simulink model "traffic_light_with_urgent_manger_B2B"  (R2020a)
settings: Solver=VariableStepAuto  StartTime=0.0  StopTime=10.0  RelTol=1e-3
libraries: pil_lib x1
settings Model: Creator=Administrator  LastModifiedBy=Administrator

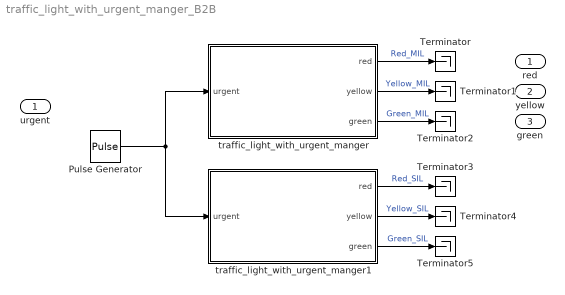
== system traffic_light_with_urgent_manger_B2B ==
  urgent : Inport
  Pulse Generator : DiscretePulseGenerator  PulseType=Time based  Period=10  PulseWidth=5
  Terminator{,1..5} (6 alike) : Terminator
  traffic_light_with_urgent_manger : Stateflow chart  TreatAsAtomicUnit=on
  traffic_light_with_urgent_manger1 : Subsystem  Tag=__SL_testing_harness_stub_  DialogController=pil_create_dialog  LoadFcn=|
      | try
      |    if ~strcmp(rtw.pil.getPILVersion, '9.8 (R2020a)_13')
      |       set_param(gcb, 'DialogController', '');
      |       set_param(gcb, 'DialogControllerArgs', '');
      |    end
      | catch e
      |       set_param(gcb, 'DialogController', '');
      |       set_param(gcb, 'DialogControllerArgs', '');
      | end
      mask help: PIL:pil:XILBlockMaskDesc
      mask Display: disp('SIL');
  red : Outport
  yellow : Outport  Port=2
  green : Outport  Port=3
  wires:
  Pulse Generator/1 -> traffic_light_with_urgent_manger1/1(urgent), traffic_light_with_urgent_manger/1(urgent)
  traffic_light_with_urgent_manger/1(red) -> Terminator/1  "Red_MIL"
  traffic_light_with_urgent_manger/2(yellow) -> Terminator1/1  "Yellow_MIL"
  traffic_light_with_urgent_manger/3(green) -> Terminator2/1  "Green_MIL"
  traffic_light_with_urgent_manger1/1(red) -> Terminator3/1  "Red_SIL"
  traffic_light_with_urgent_manger1/2(yellow) -> Terminator4/1  "Yellow_SIL"
  traffic_light_with_urgent_manger1/3(green) -> Terminator5/1  "Green_SIL"

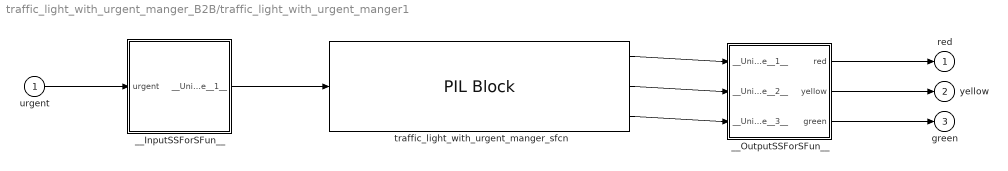
== system traffic_light_with_urgent_manger_B2B/traffic_light_with_urgent_manger1 ==
  urgent : Inport
  __InputSSForSFun__ : Subsystem
  __OutputSSForSFun__ : Subsystem
  traffic_light_with_urgent_manger_sfcn : pil_lib/PIL Block  SimulationMode=SIL  IsTopModelPIL=off  CodeDir=C:\Users\Administrator\Desktop\2020m\state_flow\1\traffic_light_with_urgent_manger\traffic_light_with_urgent_mange_ert_rtw  AnchorDir=C:\Users\Administrator\Desktop\2020m\state_flow\1\traffic_light_with_urgent_manger  ConfigName=Software-in-the-Loop (SIL)  XrelIsTopModelCode=on  XrelIsReusable=off  XrelDWorkNames={}  XrelDWorkTypes={}  XrelModelArgVals={}  XrelOrderedParamNames={}
      settings: SourceProductBaseCode=RT
  red : Outport
  yellow : Outport  Port=2
  green : Outport  Port=3
  wires:
  __OutputSSForSFun__/3(green) -> green/1
  __OutputSSForSFun__/2(yellow) -> yellow/1
  __OutputSSForSFun__/1(red) -> red/1
  traffic_light_with_urgent_manger_sfcn/3 -> __OutputSSForSFun__/3(__UniqueInportName__3__)
  traffic_light_with_urgent_manger_sfcn/2 -> __OutputSSForSFun__/2(__UniqueInportName__2__)
  traffic_light_with_urgent_manger_sfcn/1 -> __OutputSSForSFun__/1(__UniqueInportName__1__)
  __InputSSForSFun__/1(__UniqueOutportName__1__) -> traffic_light_with_urgent_manger_sfcn/1
  urgent/1 -> __InputSSForSFun__/1(urgent)

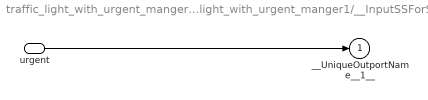
== system traffic_light_with_urgent_manger_B2B/traffic_light_with_urgent_manger1/__InputSSForSFun__ ==
  urgent : Inport
  __UniqueOutportName__1__ : Outport
  wires:
  urgent/1 -> __UniqueOutportName__1__/1

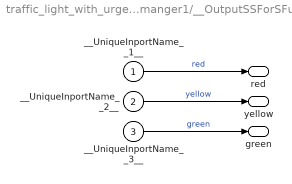
== system traffic_light_with_urgent_manger_B2B/traffic_light_with_urgent_manger1/__OutputSSForSFun__ ==
  __UniqueInportName__1__ : Inport
  __UniqueInportName__2__ : Inport  Port=2
  __UniqueInportName__3__ : Inport  Port=3
  red : Outport
  yellow : Outport  Port=2
  green : Outport  Port=3
  wires:
  __UniqueInportName__3__/1 -> green/1  "green"
  __UniqueInportName__2__/1 -> yellow/1  "yellow"
  __UniqueInportName__1__/1 -> red/1  "red"

== stateflow chart traffic_light_with_urgent_manger_B2B/traffic_light_with_urgent_manger ==
  state normal
    state stop
      en:
      red=1;
      ex:
      red=0;
    state ready
      en:
      yellow=1;
      ex:
      yellow=0;
    state go
      en:
      green=1;
      ex:
      green=0;
    (default) -> normal.stop
    go -> normal.stop : after(1,sec)
    normal.stop -> ready : after(1,sec)
    ready -> go : after(1,sec)
  state fault
    state stop
      en:
      red=1;
      ex:
      red=0;
    state start
      en:
      red=0;
      ex:
      red=0;
    (default) -> fault.stop
    fault.stop -> start : [urgent==0]
  (default) -> normal
  normal -> fault : [urgent==1]
  fault -> normal : [urgent==0]
  data: urgent input; red output; yellow output; green output
